simulink library "ScalarChimeControlLib"  (R2022b)
settings: Solver=VariableStepAuto  StartTime=0.0  StopTime=10.0  RelTol=1e-3
values from neighbouring files (symbols this model uses):
  gain = chimeConfig.rgainz.gain    [chimes_init.m]
  nch = Nch    (= 1)    [chimes_init.m]
  OffsetIntChime = 1    [ChimeControlConfig.m]
  SelectNumIntChimes = [1 2 3 4]    [ChimeControlConfig.m]
  sysin_channel_count = chimeConfig.rgainz.sysin_channel_count    [chimes_init.m]
undefined symbols (not defined in the file or in its folder): CHECK_GROUP_COUNT, CHECK_PULSE_COUNT, chime_input_index, chimeCancel, CHIMECONTROL_NSTATES, chimeEndNotification, chimePlayPending, chimeRouting, chimeType, count, countDecrement, countState, decrementVals, endOfFinalChime, FALL, fallTime, forever, FW_AppendHostNotification, IDLE, immediately, include_internal_chime_flag, include_internal_click_clack, newProfile, nextState_expired, nextState_notExpired, nInternalBeepsGongs, NSTATES, num_chime_count, num_click_clack, num_external_chime, num_inp_chs, num_internal_chime, numPulses, offTime, onTime, outputState, period, playback_flag, remainingCount, RISE, riseTime, RTC_SIM_OBJ, spkrRouting, startOfFinalChime, state, sys_defs, thresholdNumPulse, volume, WAIT_FOR_PERIOD
libraries: ScalarChimeControlLibBtc x1
settings Model: Creator=nikunj.tapodhan  LastModifiedBy=kl13806
settings SolverCC: AlgebraicLoopSolver=TrustRegion
settings DebuggingCC: UnconnectedInputMsg=warning  UnconnectedOutputMsg=warning  UnconnectedLineMsg=warning  SFMachineParentedDataDiag=warning  ArithmeticOperatorsInVariantConditions=warning
settings ModelReferenceCC: EnableRefExpFcnMdlSchedulingChecks=on
settings SFSimCC: CustomCodeUndefinedFunction=UseInterfaceOnly
settings RTWCC: DLArmComputeVersion=19.05

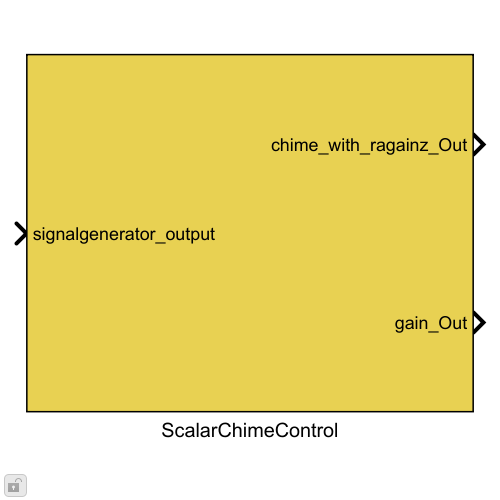
[thumbnail: Simulink's stored preview of the top-level diagram]
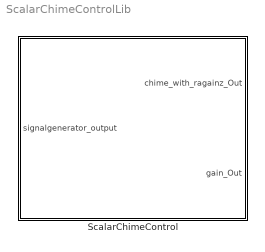
== system ScalarChimeControlLib ==
  ScalarChimeControl : Subsystem  mask{Fs_Hz=sys_defs.Fs_Hz, frameSize_samples=sys_defs.frameSize_samples, sineTableLength=sys_defs.sineTableLength, num_internal_chime=num_internal_chime, num_external_chime=num_external_chime, num_click_clack=num_click_clack, include_internal_chime_flag=include_internal_chime_flag, nch=nch, num_inp_chs=num_inp_chs, NSTATES=NSTATES, decrementVals=decrementVals, count=count, countDecrement=countDecrement, state=state, countState=countState, nextState_expired=nextState_expired, nextState_notExpired=nextState_notExpired, outputState=outputState, IDLE=IDLE, RISE=RISE, FALL=FALL, CHECK_PULSE_COUNT=CHECK_PULSE_COUNT, WAIT_FOR_PERIOD=WAIT_FOR_PERIOD, CHECK_GROUP_COUNT=CHECK_GROUP_COUNT, CHIMECONTROL_NSTATES=CHIMECONTROL_NSTATES, volume=volume, riseTime=riseTime, onTime=onTime, fallTime=fallTime, offTime=offTime, numPulses=numPulses, period=period, startOfFinalChime=startOfFinalChime, endOfFinalChime=endOfFinalChime, chimeEndNotification=chimeEndNotification, newProfile=newProfile, chimeRouting=chimeRouting, num_chime_count=num_chime_count, spkrRouting=spkrRouting, chimePlayPending=chimePlayPending, remainingCount=remainingCount, FW_AppendHostNotification=FW_AppendHostNotification, chimeCancel=chimeCancel, chimeType=chimeType, nInternalBeepsGongs=nInternalBeepsGongs, chime_input_index=chime_input_index, include_internal_click_clack=include_internal_click_clack, thresholdNumPulse=thresholdNumPulse, OffsetIntChime=OffsetIntChime, SelectNumIntChimes=SelectNumIntChimes, immediately=immediately, forever=forever, playback_flag=playback_flag, RTC_SIM_OBJ=RTC_SIM_OBJ, sysin_channel_count=sysin_channel_count, gain=gain}
      mask prompts: sysin_channel_count "Number of rampers"; gain "Initial ramper gains"
      mask init:
      | blkh = gcbh;
      | % Copy discrete mask parameters into a classdef object
      | InnerLinkConfig = ScalarChimeControlConfig;
      | InnerLinkConfig.FsHz = Fs_Hz;
      | InnerLinkConfig.FrameSizeSamples = frameSize_samples;
      | InnerLinkConfig.SineTableLength = sineTableLength;
      | InnerLinkConfig.NumInternalChime = num_internal_chime;
      | % InnerLinkConfig.NumExternalChime = num_external_chime;
      | InnerLinkConfig.NumClickClack = num_click_clack;
      | InnerLinkConfig.IncludeInternalChimeFlag = include_internal_chime_flag;
      | InnerLinkConfig.Nch = nch;
      | InnerLinkConfig.NumInpChs = num_inp_chs;
      | InnerLinkConfig.NStates = NSTATES;
      | InnerLinkConfig.DecrementVals = decrementVals;
      | InnerLinkConfig.Count = count;
      | InnerLinkConfig.CountDecrement = countDecrement;
      | InnerLinkConfig.State = state;
      | InnerLinkConfig.CountState = countState;
      | InnerLinkConfig.NextStateExpired = nextState_expired;
      | InnerLinkConfig.NextStateNotExpired = nextState_notExpired;
      | InnerLinkConfig.OutputState = outputState;
      | InnerLinkConfig.Idle = IDLE;
      | InnerLinkConfig.Rise = RISE;
      | InnerLinkConfig.Fall = FALL;
      | InnerLinkConfig.CheckPulseCount = CHECK_PULSE_COUNT;
      | InnerLinkConfig.WaitForPeriod = WAIT_FOR_PERIOD;
      | InnerLinkConfig.CheckGroupCount = CHECK_GROUP_COUNT;
      | InnerLinkConfig.ChimecontrolNstates = CHIMECONTROL_NSTATES;
      | InnerLinkConfig.Volume = volume;
      | InnerLinkConfig.RiseTime = riseTime;
      | InnerLinkConfig.OnTime = onTime;
      | InnerLinkConfig.FallTime = fallTime;
      | InnerLinkConfig.OffTime = offTime;
      | InnerLinkConfig.NumPulses = numPulses;
      | InnerLinkConfig.Period = period;
      | InnerLinkConfig.StartOfFinalChime = startOfFinalChime;
      | InnerLinkConfig.EndOfFinalChime = endOfFinalChime;
      | InnerLinkConfig.ChimeEndNotification = chimeEndNotification;
      | InnerLinkConfig.NewProfile = newProfile;
      | InnerLinkConfig.ChimeRouting = chimeRouting;
      | InnerLinkConfig.NumChimeCount = num_chime_count;
      | % InnerLinkConfig.SpkrRouting = spkrRouting;
      | InnerLinkConfig.ChimePlayPending = chimePlayPending;
      | InnerLinkConfig.RemainingCount = remainingCount;
      | InnerLinkConfig.FwAppendHostNotification = FW_AppendHostNotification;
      | InnerLinkConfig.ChimeCancel = chimeCancel;
      | InnerLinkConfig.ChimeType = chimeType;
      | InnerLinkConfig.NInternalBeepsGongs = nInternalBeepsGongs;
      | InnerLinkConfig.ChimeInputIndex = chime_input_index;
      | InnerLinkConfig.IncludeInternalClickClack = include_internal_click_clack;
      | InnerLinkConfig.ThresholdNumPulse = thresholdNumPulse;
      | InnerLinkConfig.OffsetIntChime = OffsetIntChime;
      | InnerLinkConfig.SelectNumIntChimes = SelectNumIntChimes;
      | InnerLinkConfig.Immediately = immediately;
      | InnerLinkConfig.Forever = forever;
      | InnerLinkConfig.PlaybackFlag = playback_flag;
      | InnerLinkConfig.SysInChannelCount = sysin_channel_count;
      | InnerLinkConfig.Gain = gain;

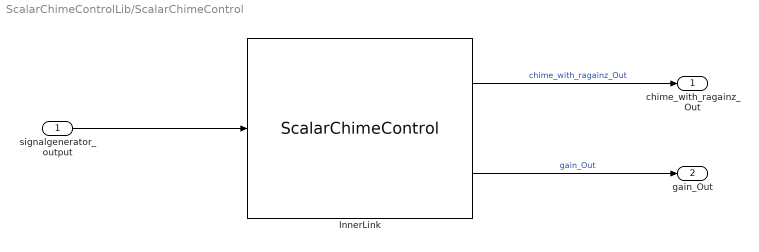
== system ScalarChimeControlLib/ScalarChimeControl ==
  signalgenerator_output : Inport
  InnerLink : ScalarChimeControlLibBtc/ScalarChimeControl  Config=InnerLinkConfig
      settings: SourceProductName=Bose Blocklib
  chime_with_ragainz_Out : Outport
  gain_Out : Outport  Port=2
  wires:
  InnerLink/1 -> chime_with_ragainz_Out/1  "chime_with_ragainz_Out"
  InnerLink/2 -> gain_Out/1  "gain_Out"
  signalgenerator_output/1 -> InnerLink/1
